simulink model "VehCtrlMdel240918_2018b"  (R2019b)
settings: Solver=FixedStepDiscrete  StartTime=0.0  StopTime=10.0  FixedStep=0.0005  RelTol=1e-3  EnableMultiTasking=on
values from neighbouring files (symbols this model uses):
  Ax_OffSet = 0.0    [VehCtrlMdelDictionary.sldd]
  Ay_OffSet = 0.0    [VehCtrlMdelDictionary.sldd]
  Caf = 460.0    [VehCtrlMdelDictionary.sldd]    (also in trqvparameter.m = 460)
  Car = 440.0    [VehCtrlMdelDictionary.sldd]    (also in trqvparameter.m = 440)
  dwf = 1.2    [VehCtrlMdelDictionary.sldd]    (also in trqvparameter.m)
  dwr = 1.2    [VehCtrlMdelDictionary.sldd]    (also in trqvparameter.m)
  h = 0.29    [VehCtrlMdelDictionary.sldd]    (also in trqvparameter.m)
  i1 = 11.4    [VehCtrlMdelDictionary.sldd]    (also in trqvparameter.m)
  i2 = 3.4    [VehCtrlMdelDictionary.sldd]    (also in trqvparameter.m)
  Iz = 105.0    [VehCtrlMdelDictionary.sldd]    (also in trqvparameter.m = 105)
  Kc = 1.0    [VehCtrlMdelDictionary.sldd]    (also in trqvparameter.m = 10)
  Ki = 1.0    [VehCtrlMdelDictionary.sldd]    (also in trqvparameter.m = 20)
  Kp = 2.0    [VehCtrlMdelDictionary.sldd]    (also in trqvparameter.m = 30)
  Ldwf = 1.2    [VehCtrlMdelDictionary.sldd]    (also in trqvparameter.m)
  Ldwr = 1.16    [VehCtrlMdelDictionary.sldd]    (also in trqvparameter.m)
  lf = 0.761    [VehCtrlMdelDictionary.sldd]    (also in trqvparameter.m)
  lr = 0.831    [VehCtrlMdelDictionary.sldd]    (also in trqvparameter.m)
  m = 340.0    [VehCtrlMdelDictionary.sldd]    (also in trqvparameter.m = 340)
  Offset_Angle = 0.0    [VehCtrlMdelDictionary.sldd]
  Qa = 0.1    [VehCtrlMdelDictionary.sldd]    (also in trqvparameter.m)
  Ra = 2.0    [VehCtrlMdelDictionary.sldd]    (also in trqvparameter.m = 2)
  Rt = 0.2    [VehCtrlMdelDictionary.sldd]    (also in trqvparameter.m)
  thr1 = 2.0    [VehCtrlMdelDictionary.sldd]    (also in trqvparameter.m = 2)
  thr2 = 0.5    [VehCtrlMdelDictionary.sldd]    (also in trqvparameter.m)
  thr3 = 0.8    [VehCtrlMdelDictionary.sldd]    (also in trqvparameter.m)
  thr4 = 0.5    [VehCtrlMdelDictionary.sldd]    (also in trqvparameter.m)
  thr5 = -0.5    [VehCtrlMdelDictionary.sldd]    (also in trqvparameter.m)
  TrqRquRate = 0.1    [VehCtrlMdelDictionary.sldd]    (also in trqvparameter.m)
  YawRate_OffSet = 0.0    [VehCtrlMdelDictionary.sldd]
undefined symbols (not defined in the file or in its folder): DiscIntNeverNeededParam, I_AN07_5V, I_AN08_5V, I_AN09_5V, I_AN10_5V, I_SW01_L, I_SW02_L, I_SW03_L, O_SW12_HS1A, O_SW14_HS1A, PWM3
libraries: simulink x144, ec5744lib x68, canmsglib x18
(part 3 of 5)

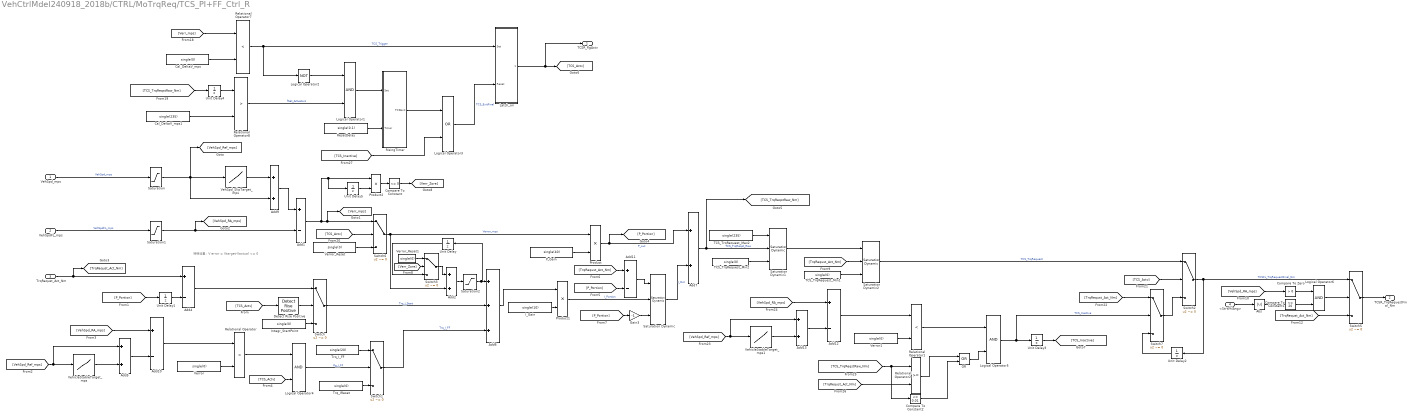
== system VehCtrlMdel240918_2018b/CTRL/MoTrqReq/TCS_PI+FF_Ctrl_R ==
  note: 特殊设置：V error = Vtarget-Vactual <= 0
  VehSpd_mps : Inport
  VehSpdFL_mps : Inport  Port=2
  TrqRequst_Act_Nm : Inport  Port=3
  <StrWhlAng> : Inport  Port=4
  Abs : Abs
  Add{1,4,10..12} (5 alike) : Sum  Inputs=+-
  Add{2,5,7,9,13} (5 alike) : Sum
  Add6 : Sum  Inputs=+++
  Cal_DeltaV_mps : Constant  Value=single(0)
  Cal_DeltaV_mps1 : Constant  Value=single(235)
  Compare To Constant : simulink/Logic and Bit Operations/Compare To Constant  relop=<=  const=0  OutDataTypeStr=boolean
  Compare To Constant1 : simulink/Logic and Bit Operations/Compare To Constant  relop=<=  const=20  OutDataTypeStr=boolean
  Compare To Constant2 : simulink/Logic and Bit Operations/Compare To Constant  relop=<=  const=0.01  OutDataTypeStr=boolean
  Compare To Zero : simulink/Logic and Bit Operations/Compare To Zero  relop=>  OutDataTypeStr=boolean
  Detect Rise Positive : simulink/Logic and Bit Operations/Detect Rise Positive  vinit=0  OutDataTypeStr=boolean
  Gain3 : Gain  Gain=-1
  I_Gain : Constant  Value=single(10)
  Integr_StartPoint : Constant  Value=single(0)
  Latch_on : Subsystem
  Logical Operator{1,4..6} (4 alike) : Logic  AllPortsSameDT=off  OutDataTypeStr=boolean
  Logical Operator2 : Logic  Operator=NOT  AllPortsSameDT=off  OutDataTypeStr=boolean
  Logical Operator3 : Logic  Operator=OR  AllPortsSameDT=off  OutDataTypeStr=boolean
  OR : Logic  Operator=OR  AllPortsSameDT=off  OutDataTypeStr=boolean
  P_Gain : Constant  Value=single(40)
  Product : Product
  Product1 : Product
  Product2 : Product
  Relational Operator : RelationalOperator  Operator=<  OutDataTypeStr=boolean  RndMeth=Simplest
  Relational Operator1 : RelationalOperator  Operator=<  OutDataTypeStr=boolean  RndMeth=Simplest
  Relational Operator2 : RelationalOperator  OutDataTypeStr=boolean  RndMeth=Simplest
  Relational Operator7 : RelationalOperator  Operator=<  OutDataTypeStr=boolean  RndMeth=Simplest
  Relational Operator8 : RelationalOperator  Operator=>  OutDataTypeStr=boolean  RndMeth=Simplest
  ResetDelay : Constant  Value=single(0.1)
  RisingTimer : Subsystem
  Saturation : Saturate  UpperLimit=40  LowerLimit=0
  Saturation Dynamic : simulink/Discontinuities/Saturation Dynamic  OutMin=[]  OutMax=[]  OutDataTypeStr=Inherit: Same as second input  OutDataType=fixdt(1, 16)  OutScaling=2^-10  DoSatur=off
  Saturation Dynamic1 : simulink/Discontinuities/Saturation Dynamic  OutMin=[]  OutMax=[]  OutDataTypeStr=Inherit: Same as second input  OutDataType=fixdt(1, 16)  OutScaling=2^-10  DoSatur=off
  Saturation Dynamic2 : simulink/Discontinuities/Saturation Dynamic  OutMin=[]  OutMax=[]  OutDataTypeStr=Inherit: Same as second input  OutDataType=fixdt(1, 16)  OutScaling=2^-10  DoSatur=off
  Saturation1 : Saturate  UpperLimit=50  LowerLimit=0
  Saturation2 : Saturate  UpperLimit=400  LowerLimit=-100
  Switch{,1..3,5..7} (7 alike) : Switch  Criteria=u2 ~= 0
  TCS_TrqRequest_Max2 : Constant  Value=single(235)
  TCS_TrqRequest_Min1 : Constant  Value=single(0)
  TCS_TrqRequest_Min2 : Constant  Value=single(0)
  Trq_IReset : Constant  Value=single(0)
  Trq_I_FF : Constant  Value=single(20)
  Unit Delay{,1..5} (6 alike) : UnitDelay  SampleTime=-1  HasFrameUpgradeWarning=on
  VehSpd_SlipTarget_mps : Lookup_n-D  NumberOfTableDimensions=1  BreakpointsForDimension1=[0,3,25,30]  Table=[0.3,0.3,2.5,2.5]  ExtrapMethod=Clip  InternalRulePriority=Speed  RndMeth=Simplest  InputSameDT=on
  VehicleStableTarget_mps : Lookup_n-D  NumberOfTableDimensions=1  BreakpointsForDimension1=[0,3,25,30]  Table=[0.4,0.4,1.2,1.2]  ExtrapMethod=Clip  InternalRulePriority=Speed  RndMeth=Simplest  InputSameDT=on
  VehicleStableTarget_mps1 : Lookup_n-D  NumberOfTableDimensions=1  BreakpointsForDimension1=[0,3,25,30]  Table=[0.4,0.4,1.2,1.2]  ExtrapMethod=Clip  InternalRulePriority=Speed  RndMeth=Simplest  InputSameDT=on
  Verror : Constant  Value=single(0)
  Verror1 : Constant  Value=single(0)
  Verror_Reset : Constant  Value=single(0)
  Verror_Reset1 : Constant  Value=single(0)
  TCSR_flgActv : Outport
  TCSR_TrqRequestFinal_Nm : Outport  Port=2
  wires:
  Add1/1 -> Unit Delay5/1, Product2/1, Switch6/1, [Verr_mps]
  Switch2/1 -> Switch5/1, Unit Delay2/1  "TCSFL_TrqRequestFinal_Nm"
  Saturation/1 -> Add9/2, VehSpd_SlipTarget_mps/1, [VehSpd_Ref_mps]
  Gain3/1 -> Saturation Dynamic/3
  [P_Portion] -> Gain3/1
  P_Gain/1 -> Product/2
  Unit Delay/1 -> Switch3/3
  Add2/1 -> Saturation2/1
  [TrqRequst_Act_Nm] -> Add11/1
  Saturation2/1 -> Unit Delay/1, Add6/1
  Switch/1 -> Add6/2  "Trq_I_Start"
  Saturation Dynamic/1 -> Add7/2  "I_Out"
  VehSpd_mps/1 -> Saturation/1  "VehSpd_mps"
  Saturation1/1 -> Add1/2, [VehSpd_RA_mps]
  Product1/1 -> Saturation Dynamic/2  "I_Portion"
  TrqRequst_Act_Nm/1 -> Add4/1, [TrqRequst_Act_Nm]
  Add6/1 -> Product1/1
  TCS_TrqRequest_Min1/1 -> Saturation Dynamic2/3
  Detect Rise Positive/1 -> Switch/2
  Integr_StartPoint/1 -> Switch/3
  I_Gain/1 -> Product1/2
  Saturation Dynamic2/1 -> Switch2/1  "TCS_TrqRequest"
  Add7/1 -> Saturation Dynamic1/2, [TCS_TrqReqstRaw_Nm]  "TCS_TrqReqst_Raw"
  [TrqRequst_Act_Nm] -> Saturation Dynamic2/2
  VehSpd_SlipTarget_mps/1 -> Add9/1
  Add9/1 -> Add1/1
  [Verr_mps] -> Relational Operator7/1
  Cal_DeltaV_mps/1 -> Relational Operator7/2
  Relational Operator7/1 -> Latch_on/1(Set), Logical Operator2/1  "TCS_Trigger"
  [TCS_TrqReqstRaw_Nm] -> Unit Delay4/1
  Logical Operator2/1 -> Logical Operator1/1
  Relational Operator8/1 -> Logical Operator1/2  "fSat_Actuators"
  Cal_DeltaV_mps1/1 -> Relational Operator8/2
  Logical Operator1/1 -> RisingTimer/1(Set)
  ResetDelay/1 -> RisingTimer/2(Timer)
  RisingTimer/1(TCSExit) -> Logical Operator3/1
  Logical Operator3/1 -> Latch_on/2(Reset)  "TCS_ExitFinal"
  Latch_on/1(flg_TCSActv) -> TCSR_flgActv/1, [TCS_Actv]
  [TCS_Actv] -> Switch6/2
  Verror_Reset/1 -> Switch6/3
  Switch6/1 -> Product/1, Add2/2  "Verror_mps"
  Product/1 -> [P_Portion], Add7/1  "P_out"
  [TCS_Actv] -> Detect Rise Positive/1
  [P_Portion] -> Unit Delay1/1
  Add4/1 -> Switch/1
  Unit Delay1/1 -> Add4/2
  [VehSpd_Ref_mps] -> Add5/1, VehicleStableTarget_mps/1
  VehicleStableTarget_mps/1 -> Add5/2
  Add5/1 -> Add10/2
  [VehSpd_RA_mps] -> Add10/1
  Add10/1 -> Relational Operator/1
  Verror/1 -> Relational Operator/2
  Relational Operator/1 -> Logical Operator4/1
  [TCS_Actv] -> Logical Operator4/2
  Logical Operator4/1 -> Switch1/2  "flg_I_FF"
  Trq_I_FF/1 -> Switch1/1
  Trq_IReset/1 -> Switch1/3
  Switch1/1 -> Add6/3  "Trq_I_FF"
  [P_Portion] -> Add11/2
  Add11/1 -> Saturation Dynamic/1
  [TCS_Actv] -> Switch2/2
  Switch7/1 -> Switch2/3
  [TrqRequst_Act_Nm] -> Switch7/1
  Verror1/1 -> Relational Operator1/2
  Add12/1 -> Relational Operator1/1
  [VehSpd_RA_mps] -> Add12/1
  Add13/1 -> Add12/2
  VehicleStableTarget_mps1/1 -> Add13/2
  [VehSpd_Ref_mps] -> VehicleStableTarget_mps1/1, Add13/1
  [TCS_TrqReqstRaw_Nm] -> Compare To Constant2/1, Relational Operator2/1
  [TrqRequst_Act_Nm] -> Relational Operator2/2
  Relational Operator1/1 -> Logical Operator5/1
  Relational Operator2/1 -> OR/1
  Logical Operator5/1 -> Unit Delay3/1, Switch7/2  "TCS_Inactive"
  Unit Delay3/1 -> [TCS_Inactive]
  [TCS_Inactive] -> Logical Operator3/2
  Unit Delay4/1 -> Relational Operator8/1
  VehSpdFL_mps/1 -> Saturation1/1  "VehSpdFL_mps"
  Saturation Dynamic1/1 -> Saturation Dynamic2/1
  TCS_TrqRequest_Max2/1 -> Saturation Dynamic1/1
  TCS_TrqRequest_Min2/1 -> Saturation Dynamic1/3
  Switch3/1 -> Add2/1
  Verror_Reset1/1 -> Switch3/1
  [Verr_Zore] -> Switch3/2
  Unit Delay5/1 -> Product2/2
  Product2/1 -> Compare To Constant/1
  Compare To Constant/1 -> [Verr_Zore]
  <StrWhlAng>/1 -> Abs/1
  Compare To Zero/1 -> Logical Operator6/1
  Abs/1 -> Compare To Constant1/1
  [VehSpd_RA_mps] -> Compare To Zero/1
  Compare To Constant1/1 -> Logical Operator6/2
  Unit Delay2/1 -> Switch7/3
  Switch5/1 -> TCSR_TrqRequestFinal_Nm/1
  Logical Operator6/1 -> Switch5/2
  [TrqRequst_Act_Nm] -> Switch5/3
  Compare To Constant2/1 -> OR/2
  OR/1 -> Logical Operator5/2

== system VehCtrlMdel240918_2018b/Input/ABS_Receive/ABS_BUS_state ==
  CANOK : Inport
  ID : Inport  Port=2
  Msg : Inport  Port=3
  function : TriggerPort  TriggerType=function-call  VariantControl=(inherit)
  Bus Creator3 : BusCreator  Inputs=4
  IMU_state : Subsystem  TreatAsAtomicUnit=on
  ABS_BUS : Outport  VectorParamsAs1DForOutWhenUnconnected=off
  wires:
  IMU_state/3(ABS_WS_FL) -> Bus Creator3/3
  IMU_state/2(ABS_WS_RL) -> Bus Creator3/2
  IMU_state/1(ABS_WS_FR) -> Bus Creator3/1
  Bus Creator3/1 -> ABS_BUS/1
  ID/1 -> IMU_state/1(ID)
  CANOK/1 -> IMU_state/Enable
  Msg/1 -> IMU_state/2(Msg)
  IMU_state/4(ABS_WS_RR) -> Bus Creator3/4

== system VehCtrlMdel240918_2018b/Input/AMKMCU_Receive/FLAMKMCU ==
  AMKMCU_state : Subsystem  TreatAsAtomicUnit=on
  AMKMCU_state1 : Subsystem  TreatAsAtomicUnit=on
  AMKMCU_state2 : Subsystem  TreatAsAtomicUnit=on
  CANReceive1 : ec5744lib/RapidECU_U3/04CANCommunication/CANReceive  canmodule=1  canbuffer=2  canmessageid=642  canmessagetype=Standard(11-bit ID)  datalength=8  sampletime=-1
      settings: SourceProductName=ECUCoder for MPC5744
  CANReceive2 : ec5744lib/RapidECU_U3/04CANCommunication/CANReceive  canmodule=1  canbuffer=3  canmessageid=644  canmessagetype=Standard(11-bit ID)  datalength=8  sampletime=-1
      settings: SourceProductName=ECUCoder for MPC5744
  CANReceive3 : ec5744lib/RapidECU_U3/04CANCommunication/CANReceive  canmodule=1  canbuffer=1  canmessageid=640  canmessagetype=Standard(11-bit ID)  datalength=8  sampletime=-1
      settings: SourceProductName=ECUCoder for MPC5744
  Terminator1 : Terminator
  Terminator2 : Terminator
  Terminator3 : Terminator
  FLAMKMCUtoVCU1 : Outport  VectorParamsAs1DForOutWhenUnconnected=off
  FLAMKMCUtoVCU2 : Outport  Port=2  VectorParamsAs1DForOutWhenUnconnected=off
  FLAMKMCUtoVCU3 : Outport  Port=3  VectorParamsAs1DForOutWhenUnconnected=off
  wires:
  CANReceive2/2 -> AMKMCU_state2/1(CANOK)
  CANReceive1/4 -> AMKMCU_state1/3(Msg)
  CANReceive3/5 -> Terminator3/1
  CANReceive1/3 -> AMKMCU_state1/2(ID)
  CANReceive1/1 -> AMKMCU_state1/Trigger
  CANReceive2/4 -> AMKMCU_state2/3(Msg)
  CANReceive3/3 -> AMKMCU_state/2(ID)
  CANReceive3/2 -> AMKMCU_state/1(CANOK)
  CANReceive2/3 -> AMKMCU_state2/2(ID)
  CANReceive1/2 -> AMKMCU_state1/1(CANOK)
  CANReceive1/5 -> Terminator1/1
  CANReceive3/4 -> AMKMCU_state/3(Msg)
  CANReceive2/5 -> Terminator2/1
  CANReceive3/1 -> AMKMCU_state/Trigger
  CANReceive2/1 -> AMKMCU_state2/Trigger
  AMKMCU_state2/1(FLAMKMCUtoVCU3) -> FLAMKMCUtoVCU3/1  "FLAMKMCUtoVCU3"
  AMKMCU_state/1(FLAMKtoVCU1) -> FLAMKMCUtoVCU1/1
  AMKMCU_state1/1(FLAMKMCUtoVCU2) -> FLAMKMCUtoVCU2/1  "FLAMKMCUtoVCU2"

== system VehCtrlMdel240918_2018b/Input/AMKMCU_Receive/FRAMKMCU ==
  AMKMCU_state : Subsystem  TreatAsAtomicUnit=on
  AMKMCU_state1 : Subsystem  TreatAsAtomicUnit=on
  AMKMCU_state2 : Subsystem  TreatAsAtomicUnit=on
  CANReceive1 : ec5744lib/RapidECU_U3/04CANCommunication/CANReceive  canmodule=1  canbuffer=5  canmessageid=643  canmessagetype=Standard(11-bit ID)  datalength=8  sampletime=-1
      settings: SourceProductName=ECUCoder for MPC5744
  CANReceive2 : ec5744lib/RapidECU_U3/04CANCommunication/CANReceive  canmodule=1  canbuffer=6  canmessageid=387  canmessagetype=Standard(11-bit ID)  datalength=8  sampletime=-1
      settings: SourceProductName=ECUCoder for MPC5744
  CANReceive3 : ec5744lib/RapidECU_U3/04CANCommunication/CANReceive  canmodule=1  canbuffer=4  canmessageid=641  canmessagetype=Standard(11-bit ID)  datalength=8  sampletime=-1
      settings: SourceProductName=ECUCoder for MPC5744
  Terminator1 : Terminator
  Terminator2 : Terminator
  Terminator3 : Terminator
  FRAMKMCUtoVCU1 : Outport  VectorParamsAs1DForOutWhenUnconnected=off
  FRAMKMCUtoVCU2 : Outport  Port=2  VectorParamsAs1DForOutWhenUnconnected=off
  FRAMKMCUtoVCU3 : Outport  Port=3  VectorParamsAs1DForOutWhenUnconnected=off
  wires:
  AMKMCU_state1/1(FRAMKMCUtoVCU2) -> FRAMKMCUtoVCU2/1  "FRAMKMCUtoVCU2"
  AMKMCU_state/1(FRAMKMCUtoVCU1) -> FRAMKMCUtoVCU1/1  "FRAMKMCUtoVCU1"
  AMKMCU_state2/1(FRAMKMCUtoVCU3) -> FRAMKMCUtoVCU3/1  "FRAMKMCUtoVCU3"
  CANReceive2/1 -> AMKMCU_state2/Trigger
  CANReceive3/1 -> AMKMCU_state/Trigger
  CANReceive2/5 -> Terminator2/1
  CANReceive3/4 -> AMKMCU_state/3(Msg)
  CANReceive1/5 -> Terminator1/1
  CANReceive1/2 -> AMKMCU_state1/1(CANOK)
  CANReceive2/3 -> AMKMCU_state2/2(ID)
  CANReceive3/2 -> AMKMCU_state/1(CANOK)
  CANReceive3/3 -> AMKMCU_state/2(ID)
  CANReceive2/4 -> AMKMCU_state2/3(Msg)
  CANReceive1/1 -> AMKMCU_state1/Trigger
  CANReceive1/3 -> AMKMCU_state1/2(ID)
  CANReceive3/5 -> Terminator3/1
  CANReceive1/4 -> AMKMCU_state1/3(Msg)
  CANReceive2/2 -> AMKMCU_state2/1(CANOK)

== system VehCtrlMdel240918_2018b/Input/BMS_Recive/ABS_BUS_state ==
  CANOK : Inport
  ID : Inport  Port=2
  Msg : Inport  Port=3
  function : TriggerPort  TriggerType=function-call  VariantControl=(inherit)
  Bus Creator : BusCreator  Inputs=9
  IMU_state : Subsystem  TreatAsAtomicUnit=on
  BMS_BUS : Outport  VectorParamsAs1DForOutWhenUnconnected=off
  wires:
  Bus Creator/1 -> BMS_BUS/1
  ID/1 -> IMU_state/1(ID)
  CANOK/1 -> IMU_state/Enable
  Msg/1 -> IMU_state/2(Msg)
  IMU_state/1(BatAlmlv) -> Bus Creator/1
  IMU_state/2(BatLife) -> Bus Creator/2
  IMU_state/3(BatState) -> Bus Creator/3
  IMU_state/4(LSBAz) -> Bus Creator/4
  IMU_state/5(LSBVz) -> Bus Creator/5
  IMU_state/6(MSBAz) -> Bus Creator/6
  IMU_state/7(MSBVz) -> Bus Creator/7
  IMU_state/8(SOCz) -> Bus Creator/8
  IMU_state/9(SOHz) -> Bus Creator/9

== system VehCtrlMdel240918_2018b/Input/EMRAXMCU_RECIEVE/MCU_pwr ==
  CANOK : Inport
  ID : Inport  Port=2
  Msg : Inport  Port=3
  function : TriggerPort  TriggerType=function-call  VariantControl=(inherit)
  Bus Creator3 : BusCreator  Inputs=5
  MCU_VCUMeter1 : Subsystem  TreatAsAtomicUnit=on
  MCU_pwr : Outport
  wires:
  Bus Creator3/1 -> MCU_pwr/1
  Msg/1 -> MCU_VCUMeter1/2(Msg)
  CANOK/1 -> MCU_VCUMeter1/Enable
  ID/1 -> MCU_VCUMeter1/1(ID)
  MCU_VCUMeter1/1("AC_current ") -> Bus Creator3/1  "AC_current"
  MCU_VCUMeter1/2(MCU_temp) -> Bus Creator3/2  "MCU_temp"
  MCU_VCUMeter1/3(current) -> Bus Creator3/3  "current"
  MCU_VCUMeter1/4(motor_temp) -> Bus Creator3/4  "motor_temp"
  MCU_VCUMeter1/5(voltage) -> Bus Creator3/5  "voltage"

== system VehCtrlMdel240918_2018b/Input/EMRAXMCU_RECIEVE/MCU_state ==
  CANOK : Inport
  ID : Inport  Port=2
  Msg : Inport  Port=3
  function : TriggerPort  TriggerType=function-call  VariantControl=(inherit)
  Bus Creator3 : BusCreator  Inputs=15
  MCU_state : Subsystem  TreatAsAtomicUnit=on
  Out1 : Outport  VectorParamsAs1DForOutWhenUnconnected=off
  wires:
  Msg/1 -> MCU_state/2(Msg)
  CANOK/1 -> MCU_state/Enable
  ID/1 -> MCU_state/1(ID)
  Bus Creator3/1 -> Out1/1
  MCU_state/1(12V_error) -> Bus Creator3/1
  MCU_state/2(alarm) -> Bus Creator3/2
  MCU_state/3(undervol) -> Bus Creator3/3
  MCU_state/4(controller_ready) -> Bus Creator3/4
  MCU_state/5(MCU_temp_warn) -> Bus Creator3/5
  MCU_state/6(mode_cmd8) -> Bus Creator3/6
  MCU_state/7(motor_temp_warn) -> Bus Creator3/7
  MCU_state/8(overcur) -> Bus Creator3/8
  MCU_state/9(pow_lim_warn) -> Bus Creator3/9
  MCU_state/10(overvol) -> Bus Creator3/10
  MCU_state/11(precharge) -> Bus Creator3/11
  MCU_state/12(rotation_warn) -> Bus Creator3/12
  MCU_state/13(selfcech) -> Bus Creator3/13
  MCU_state/14(RPM) -> Bus Creator3/14
  MCU_state/15(torque) -> Bus Creator3/15

== system VehCtrlMdel240918_2018b/Input/IMU_Recieve/IMU_state ==
  CANOK : Inport
  ID : Inport  Port=2
  Msg : Inport  Port=3
  function : TriggerPort  TriggerType=function-call  VariantControl=(inherit)
  Bus Creator3 : BusCreator  Inputs=7
  MCU_state : Subsystem  TreatAsAtomicUnit=on
  MeaModule1 : ec5744lib/RapidECU_U3/07Calibration/MeaModule  signal=IMU_Ax_Value
      settings: SourceProductName=ECUCoder for MPC5744
  IMU_BUS : Outport  VectorParamsAs1DForOutWhenUnconnected=off
  wires:
  Msg/1 -> MCU_state/2(Msg)
  CANOK/1 -> MCU_state/Enable
  ID/1 -> MCU_state/1(ID)
  Bus Creator3/1 -> IMU_BUS/1
  MeaModule1/1 -> Bus Creator3/1
  MCU_state/2(IMU_Ay_Value) -> Bus Creator3/2  "IMU_Ay_Value"
  MCU_state/3(IMU_Yaw_Value) -> Bus Creator3/3  "IMU_Yaw_Value"
  MCU_state/4(IMU_Ay_Valid) -> Bus Creator3/4  "IMU_Ay_Valid"
  MCU_state/5(IMU_DTC) -> Bus Creator3/5  "IMU_DTC"
  MCU_state/6(IMU_Yaw_Valid) -> Bus Creator3/6  "IMU_Yaw_Valid"
  MCU_state/7(IMU_Ax_Valid) -> Bus Creator3/7  "IMU_Ax_Valid"
  MCU_state/1(IMU_Ax_Value) -> MeaModule1/1  "IMU_Ax_Value"

== system VehCtrlMdel240918_2018b/Input/StrSnis_Receive/StrWhSnis_state ==
  CANOK : Inport
  ID : Inport  Port=2
  Msg : Inport  Port=3
  function : TriggerPort  TriggerType=function-call  VariantControl=(inherit)
  Bus Creator3 : BusCreator  Inputs=3
  IMU_state : Subsystem  TreatAsAtomicUnit=on
  IMU_BUS : Outport  VectorParamsAs1DForOutWhenUnconnected=off
  wires:
  Msg/1 -> IMU_state/2(Msg)
  CANOK/1 -> IMU_state/Enable
  ID/1 -> IMU_state/1(ID)
  Bus Creator3/1 -> IMU_BUS/1
  IMU_state/1(StrWhlAng) -> Bus Creator3/1  "StrWhlAng"
  IMU_state/2(StrWhlAngV) -> Bus Creator3/2  "StrWhlAngV"
  IMU_state/3(StrWhlAngAliveRollCnt) -> Bus Creator3/3  "StrWhlAngAliveRollCnt"

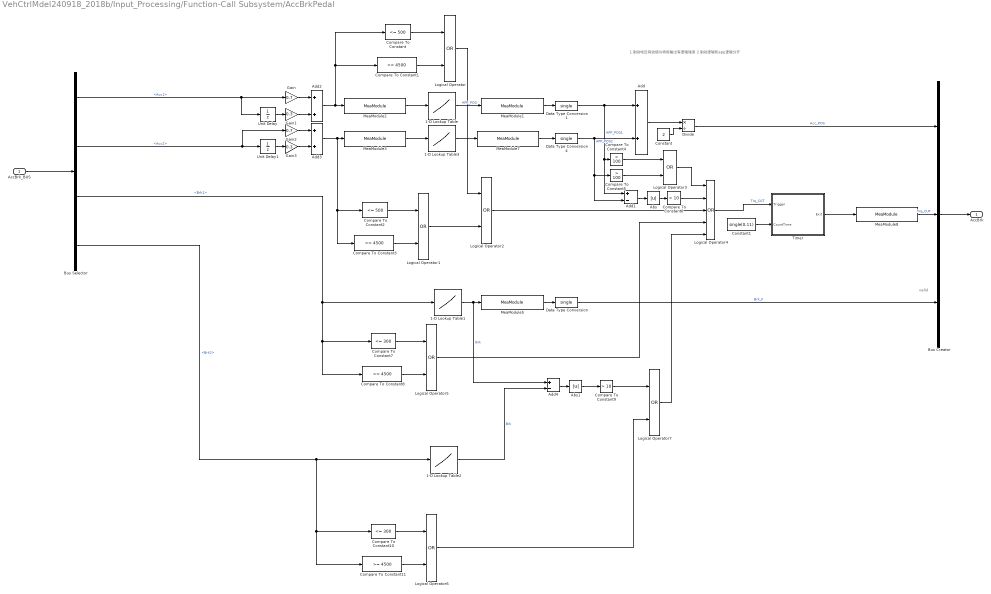
== system VehCtrlMdel240918_2018b/Input_Processing/Function-Call Subsystem/AccBrkPedal ==
  note: 1.制动电压有效值与转矩输出有逻辑错误
      | 2.制动逻辑和app逻辑分开
  note: valid
  AccBrk_BUS : Inport
  1-D Lookup Table : Lookup_n-D  NumberOfTableDimensions=1  BreakpointsForDimension1=single([1330,1590]);  BreakpointsForDimension1DataTypeStr=single  Table=single([0,100]);  TableDataTypeStr=single  ExtrapMethod=Clip  InternalRulePriority=Speed  RndMeth=Simplest  InputSameDT=on
  1-D Lookup Table1 : Lookup_n-D  NumberOfTableDimensions=1  BreakpointsForDimension1=single([500,4500]);  BreakpointsForDimension1DataTypeStr=single  Table=single([0,10000]);  TableDataTypeStr=single  ExtrapMethod=Clip  InternalRulePriority=Speed  RndMeth=Simplest  InputSameDT=on
  1-D Lookup Table2 : Lookup_n-D  NumberOfTableDimensions=1  BreakpointsForDimension1=single([500,4500]);  BreakpointsForDimension1DataTypeStr=single  Table=single([0,10000]);  TableDataTypeStr=single  ExtrapMethod=Clip  InternalRulePriority=Speed  RndMeth=Simplest  InputSameDT=on
  1-D Lookup Table3 : Lookup_n-D  NumberOfTableDimensions=1  BreakpointsForDimension1=single([2324,2600]);  BreakpointsForDimension1DataTypeStr=single  Table=single([0,100]);  TableDataTypeStr=single  ExtrapMethod=Clip  InternalRulePriority=Speed  RndMeth=Simplest  InputSameDT=on
  Abs : Abs
  Abs1 : Abs
  Add : Sum
  Add1 : Sum  Inputs=+-
  Add2 : Sum
  Add3 : Sum
  Add4 : Sum  Inputs=+-
  Bus Selector : BusSelector  OutputSignals=Acc1,Acc2,Brk1,Brk2
  Bus Creator : BusCreator  Inputs=3
  Compare To Constant : simulink/Logic and Bit Operations/Compare To Constant  relop=<=  const=500  OutDataTypeStr=boolean
  Compare To Constant{1,3,8,11} (4 alike) : simulink/Logic and Bit Operations/Compare To Constant  relop=>=  const=4500  OutDataTypeStr=boolean
  Compare To Constant10 : simulink/Logic and Bit Operations/Compare To Constant  relop=<=  const=300  OutDataTypeStr=boolean
  Compare To Constant2 : simulink/Logic and Bit Operations/Compare To Constant  relop=<=  const=500  OutDataTypeStr=boolean
  Compare To Constant4 : simulink/Logic and Bit Operations/Compare To Constant  relop=>  const=100  OutDataTypeStr=boolean
  Compare To Constant5 : simulink/Logic and Bit Operations/Compare To Constant  relop=>  const=100  OutDataTypeStr=boolean
  Compare To Constant6 : simulink/Logic and Bit Operations/Compare To Constant  relop=>  const=10  OutDataTypeStr=boolean
  Compare To Constant7 : simulink/Logic and Bit Operations/Compare To Constant  relop=<=  const=300  OutDataTypeStr=boolean
  Compare To Constant9 : simulink/Logic and Bit Operations/Compare To Constant  relop=>  const=10  OutDataTypeStr=boolean
  Constant : Constant  Value=2
  Constant1 : Constant  Value=single(0.11)
  Data Type Conversion : DataTypeConversion  OutDataTypeStr=single
  Data Type Conversion1 : DataTypeConversion  OutDataTypeStr=single
  Data Type Conversion4 : DataTypeConversion  OutDataTypeStr=single
  Divide : Product  Inputs=*/  OutDataTypeStr=single
  Gain : Gain  Gain=0.7
  Gain1 : Gain  Gain=0.3
  Gain2 : Gain  Gain=0.7
  Gain3 : Gain  Gain=0.3
  Logical Operator{,1..3,5..7} (7 alike) : Logic  Operator=OR  AllPortsSameDT=off  OutDataTypeStr=boolean
  Logical Operator4 : Logic  Operator=OR  Inputs=5  AllPortsSameDT=off  OutDataTypeStr=boolean
  MeaModule1 : ec5744lib/RapidECU_U3/07Calibration/MeaModule  signal=Acc_POS1
      settings: SourceProductName=ECUCoder for MPC5744
  MeaModule2 : ec5744lib/RapidECU_U3/07Calibration/MeaModule  signal=Acc_vol
      settings: SourceProductName=ECUCoder for MPC5744
  MeaModule3 : ec5744lib/RapidECU_U3/07Calibration/MeaModule  signal=Acc_vol2
      settings: SourceProductName=ECUCoder for MPC5744
  MeaModule5 : ec5744lib/RapidECU_U3/07Calibration/MeaModule  signal=F_BrkPrs
      settings: SourceProductName=ECUCoder for MPC5744
  MeaModule7 : ec5744lib/RapidECU_U3/07Calibration/MeaModule  signal=Acc_POS2
      settings: SourceProductName=ECUCoder for MPC5744
  MeaModule8 : ec5744lib/RapidECU_U3/07Calibration/MeaModule  signal=Trq_CUT
      settings: SourceProductName=ECUCoder for MPC5744
  Timer : Stateflow chart  TreatAsAtomicUnit=on
  Unit Delay : UnitDelay  SampleTime=-1  HasFrameUpgradeWarning=on
  Unit Delay1 : UnitDelay  SampleTime=-1  HasFrameUpgradeWarning=on
  AccBrk : Outport  VectorParamsAs1DForOutWhenUnconnected=off
  wires:
  AccBrk_BUS/1 -> Bus Selector/1
  Bus Selector/1 -> Unit Delay/1, Gain/1  "<Acc1>"
  Bus Selector/3 -> 1-D Lookup Table1/1, Compare To Constant7/1, Compare To Constant8/1  "<Brk1>"
  Bus Selector/2 -> Gain2/1, Unit Delay1/1  "<Acc2>"
  Gain/1 -> Add2/1
  Compare To Constant6/1 -> Logical Operator4/2
  Compare To Constant5/1 -> Logical Operator3/2
  Compare To Constant4/1 -> Logical Operator3/1
  Logical Operator3/1 -> Logical Operator4/1
  Unit Delay1/1 -> Gain3/1
  1-D Lookup Table/1 -> MeaModule1/1  "APP_POS"
  Gain3/1 -> Add3/2
  Add/1 -> Divide/1
  Logical Operator1/1 -> Logical Operator2/2
  Compare To Constant8/1 -> Logical Operator5/2
  Logical Operator4/1 -> Timer/1(Trigger)  "Trq_CUT"
  Logical Operator5/1 -> Logical Operator4/4
  Compare To Constant3/1 -> Logical Operator1/2
  Compare To Constant1/1 -> Logical Operator/2
  Add2/1 -> Compare To Constant/1, Compare To Constant1/1, MeaModule2/1
  Gain2/1 -> Add3/1
  Add3/1 -> Compare To Constant3/1, Compare To Constant2/1, MeaModule3/1
  1-D Lookup Table3/1 -> MeaModule7/1
  Compare To Constant7/1 -> Logical Operator5/1
  Data Type Conversion1/1 -> Add1/1, Compare To Constant4/1, Add/1  "APP_POS1"
  MeaModule8/1 -> Bus Creator/2  "Trq_CUT"
  Divide/1 -> Bus Creator/1  "Acc_POS"
  Compare To Constant/1 -> Logical Operator/1
  Constant/1 -> Divide/2
  Data Type Conversion4/1 -> Add1/2, Compare To Constant5/1, Add/2  "APP_POS2"
  MeaModule5/1 -> Data Type Conversion/1
  MeaModule3/1 -> 1-D Lookup Table3/1
  Logical Operator2/1 -> Logical Operator4/3
  Data Type Conversion/1 -> Bus Creator/3  "Brk_F"
  MeaModule2/1 -> 1-D Lookup Table/1
  Gain1/1 -> Add2/2
  Add1/1 -> Abs/1
  Abs/1 -> Compare To Constant6/1
  MeaModule7/1 -> Data Type Conversion4/1
  Compare To Constant2/1 -> Logical Operator1/1
  MeaModule1/1 -> Data Type Conversion1/1
  Logical Operator/1 -> Logical Operator2/1
  1-D Lookup Table1/1 -> Add4/1, MeaModule5/1  "Brk"
  Unit Delay/1 -> Gain1/1
  Bus Creator/1 -> AccBrk/1
  Timer/1(Exit) -> MeaModule8/1
  Constant1/1 -> Timer/2(CountTime)
  Bus Selector/4 -> Compare To Constant11/1, Compare To Constant10/1, 1-D Lookup Table2/1  "<Brk2>"
  1-D Lookup Table2/1 -> Add4/2  "Brk"
  Compare To Constant11/1 -> Logical Operator6/2
  Compare To Constant10/1 -> Logical Operator6/1
  Logical Operator6/1 -> Logical Operator7/2
  Add4/1 -> Abs1/1
  Abs1/1 -> Compare To Constant9/1
  Compare To Constant9/1 -> Logical Operator7/1
  Logical Operator7/1 -> Logical Operator4/5

== system VehCtrlMdel240918_2018b/Input_Processing/Function-Call Subsystem/IMU ==
  IMU : Inport
  Bus Selector : BusSelector  OutputSignals=IMU_Ax_Value,IMU_Ay_Value,IMU_Yaw_Value,IMU_Ay_Valid,IMU_DTC,IMU_Yaw_Valid,IMU_Ax_Valid
  Bus Creator : BusCreator  Inputs=7
  Subsystem : Subsystem
  g_mpss : Gain  Gain=9.8
  g_mpss1 : Gain  Gain=9.8
  IMU_BUS : Outport  VectorParamsAs1DForOutWhenUnconnected=off
  wires:
  IMU/1 -> Bus Selector/1
  Bus Selector/4 -> Bus Creator/4  "<IMU_Ay_Valid>"
  Bus Selector/5 -> Bus Creator/5  "<IMU_DTC>"
  Bus Selector/6 -> Bus Creator/6  "<IMU_Yaw_Valid>"
  Bus Selector/7 -> Bus Creator/7  "<IMU_Ax_Valid>"
  Bus Selector/1 -> g_mpss/1  "<IMU_Ax_Value>"
  Bus Selector/2 -> g_mpss1/1  "<IMU_Ay_Value>"
  Bus Creator/1 -> IMU_BUS/1
  g_mpss/1 -> Subsystem/1(IMU_Ax_Value)
  g_mpss1/1 -> Subsystem/2(IMU_Ay_Value)
  Bus Selector/3 -> Subsystem/3(IMU_Yaw_Value)  "<IMU_Yaw_Value>"
  Subsystem/1(IMU_Ax_Value_out) -> Bus Creator/1
  Subsystem/2(IMU_Ay_Value_out) -> Bus Creator/2
  Subsystem/3(IMU_Yaw_Value_out) -> Bus Creator/3

== system VehCtrlMdel240918_2018b/Input_Processing/Function-Call Subsystem/SWAS ==
  SWAS : Inport
  1-D Lookup Table : Lookup_n-D  NumberOfTableDimensions=1  BreakpointsForDimension1=|  Table=|  InternalRulePriority=Speed  RndMeth=Simplest  InputSameDT=on
      BreakpointsForDimension1=|
      | single([-119.993
      | -109.997
      | -100
      | -90.0034
      | -80.0067
      | -69.9933
      | -59.9966
      | -50
      | -40.0034
      | -30.0067
      | -19.9933
      | -9.99664
      | 0
      | 9.99664
      | 19.9933
      | 30.0067
      | 40.0034
      | 50
      | 59.9966
      | 69.9933
      | 80.0067
      | 90.0034
      | 100
      | 109.997
      | ]);
      Table=|
      | single([-26.072928
      | -23.62248
      | -20.834568
      | -18.002448
      | -15.197904
      | -12.620232
      | -10.131048
      | -8.139672
      | -6.2976672
      | -4.605012
      | -3.0893688
      | -1.4907528
      | -0.07467624
      | 1.40778
      | 2.9621448
      | 4.7211768
      | 6.5521152
      | 8.737056
      | 10.944144
      | 13.743144
      | 17.25012
      | 20.375424
      | 24.070536
      | 27.505584
      | ]);
  1-D Lookup Table1 : Lookup_n-D  NumberOfTableDimensions=1  BreakpointsForDimension1=|  Table=|  InternalRulePriority=Speed  RndMeth=Simplest  InputSameDT=on
      BreakpointsForDimension1=|
      | single([-119.995
      | -109.993
      | -99.9916
      | -90.0067
      | -80.005
      | -70.0034
      | -60.0017
      | -50
      | -39.9983
      | -29.9966
      | -19.995
      | -9.99328
      | 0.00840477
      | 9.99328
      | 19.995
      | 29.9966
      | 39.9983
      | 50
      | 60.0017
      | 70.0034
      | 80.005
      | 90.0067
      | 100.008
      | 109.993
      | ]);
      Table=|
      | single([-26.816256
      | -23.524848
      | -19.851048
      | -16.282584
      | -13.40676
      | -10.314792
      | -7.65504
      | -5.3554968
      | -3.4548912
      | -1.5044184
      | 0.02493504
      | 1.4379192
      | 2.8675296
      | 4.2638976
      | 5.76
      | 7.35588
      | 9.101304
      | 11.04624
      | 12.94128
      | 15.35724
      | 18.244152
      | 20.937168
      | 23.630112
      | 26.306496
      | ]);
  Abs : Abs
  Add1 : Sum
  Add2 : Sum
  Bus Selector : BusSelector  OutputSignals=StrWhlAng,StrWhlAngV
  Bus Creator : BusCreator  Inputs=5
  Compare To Constant : simulink/Logic and Bit Operations/Compare To Constant  relop=>  const=120  OutDataTypeStr=boolean
  Constant1 : Constant  Value=single(1200)
  Constant2 : Constant  Value=single(1200)
  Constant3 : Constant  Value=single(-1200)
  Constant4 : Constant  Value=single(-1200)
  Constant5 : Constant  Value=single(0.11)
  Gain : Gain  Gain=0.7
  Gain1 : Gain  Gain=0.3
  Gain2 : Gain  Gain=0.7
  Gain3 : Gain  Gain=0.3
  NOT : Logic  Operator=NOT  AllPortsSameDT=off  OutDataTypeStr=boolean
  Rate Limiter Dynamic : simulink/Discontinuities/Rate Limiter Dynamic
      settings: SourceProductName=Simulink
  Rate Limiter Dynamic1 : simulink/Discontinuities/Rate Limiter Dynamic
      settings: SourceProductName=Simulink
  Saturation1 : Saturate  UpperLimit=1200  LowerLimit=0
  Timer : Stateflow chart  TreatAsAtomicUnit=on
  Unit Delay : UnitDelay  SampleTime=-1  HasFrameUpgradeWarning=on
  Unit Delay1 : UnitDelay  SampleTime=-1  HasFrameUpgradeWarning=on
  StrWhlAng&V : Outport  VectorParamsAs1DForOutWhenUnconnected=off
  wires:
  SWAS/1 -> Bus Selector/1
  Bus Selector/2 -> Rate Limiter Dynamic1/2  "<StrWhlAngV>"
  Constant3/1 -> Rate Limiter Dynamic/3
  Constant2/1 -> Rate Limiter Dynamic/1
  Gain/1 -> Add2/1
  Gain1/1 -> Add2/2
  Rate Limiter Dynamic/1 -> Abs/1, Gain/1, Unit Delay/1
  Unit Delay/1 -> Gain1/1
  Add2/1 -> 1-D Lookup Table1/1, Bus Creator/4, 1-D Lookup Table/1  "StrWhlAng"
  Bus Creator/1 -> StrWhlAng&V/1
  Add1/1 -> Bus Creator/5  "StrWhlAngV"
  Rate Limiter Dynamic1/1 -> Saturation1/1
  Bus Selector/1 -> Rate Limiter Dynamic/2  "<StrWhlAng>"
  Constant1/1 -> Rate Limiter Dynamic1/1
  Constant4/1 -> Rate Limiter Dynamic1/3
  1-D Lookup Table/1 -> Bus Creator/2  "FLWhlStrAng"
  1-D Lookup Table1/1 -> Bus Creator/3  "FRWhlStrAng"
  Unit Delay1/1 -> Gain3/1
  Gain3/1 -> Add1/2
  Gain2/1 -> Add1/1
  Saturation1/1 -> Unit Delay1/1, Gain2/1  "StrWhlAngV"
  Abs/1 -> Compare To Constant/1
  NOT/1 -> Bus Creator/1  "WhlStrAng_Valid"
  Constant5/1 -> Timer/2(CountTime)
  Compare To Constant/1 -> Timer/1(Trigger)  "WhlStrAng_Valid"
  Timer/1(Exit) -> NOT/1

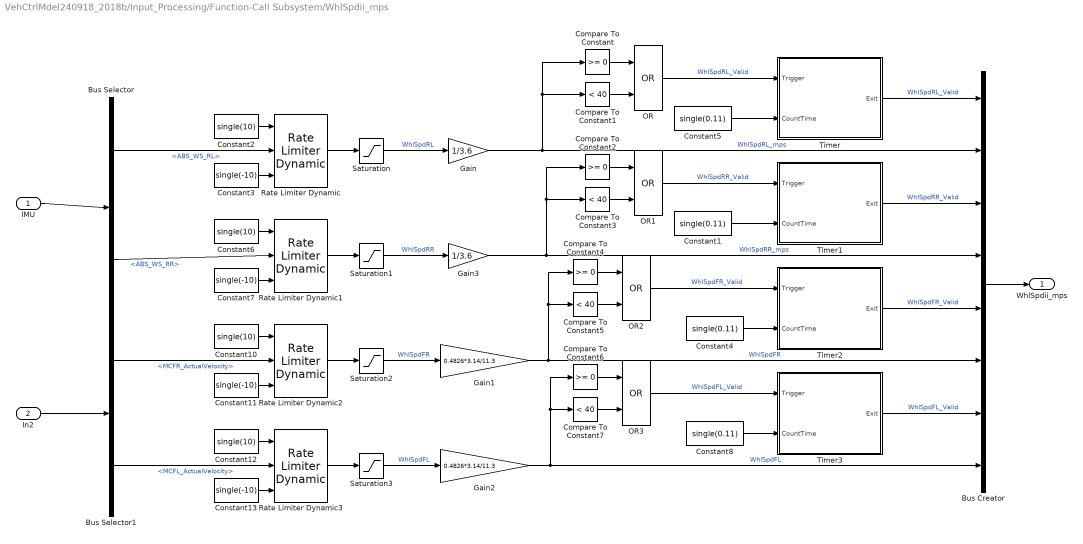
== system VehCtrlMdel240918_2018b/Input_Processing/Function-Call Subsystem/WhlSpdii_mps ==
  IMU : Inport
  In2 : Inport  Port=2
  Bus Selector : BusSelector  OutputSignals=ABS_WS_RL,ABS_WS_RR
  Bus Selector1 : BusSelector  OutputSignals=FRAMKMCUtoVCU1.MCFR_ActualVelocity,FLAMKMCUtoVCU1.MCFL_ActualVelocity
  Bus Creator : BusCreator  Inputs=8
  Compare To Constant{,2,4,6} (4 alike) : simulink/Logic and Bit Operations/Compare To Constant  relop=>=  const=0  OutDataTypeStr=boolean
  Compare To Constant{1,3,5,7} (4 alike) : simulink/Logic and Bit Operations/Compare To Constant  relop=<  const=40  OutDataTypeStr=boolean
  Constant{1,4..5,8} (4 alike) : Constant  Value=single(0.11)
  Constant{2,6,10,12} (4 alike) : Constant  Value=single(10)
  Constant{3,7,11,13} (4 alike) : Constant  Value=single(-10)
  Gain : Gain  Gain=1/3.6
  Gain1 : Gain  Gain=0.4826*3.14/11.3
  Gain2 : Gain  Gain=0.4826*3.14/11.3
  Gain3 : Gain  Gain=1/3.6
  OR{,1..3} (4 alike) : Logic  Operator=OR  AllPortsSameDT=off  OutDataTypeStr=boolean
  Rate Limiter Dynamic{,1..3} (4 alike) : simulink/Discontinuities/Rate Limiter Dynamic
      settings: SourceProductName=Simulink
  Saturation{,1..3} (4 alike) : Saturate  UpperLimit=30  LowerLimit=0
  Timer : Stateflow chart  TreatAsAtomicUnit=on
  Timer1 : Stateflow chart  TreatAsAtomicUnit=on
  Timer2 : Stateflow chart  TreatAsAtomicUnit=on
  Timer3 : Stateflow chart  TreatAsAtomicUnit=on
  WhlSpdii_mps : Outport  VectorParamsAs1DForOutWhenUnconnected=off
  wires:
  IMU/1 -> Bus Selector/1
  Bus Selector/1 -> Rate Limiter Dynamic/2  "<ABS_WS_RL>"
  Bus Selector/2 -> Rate Limiter Dynamic1/2  "<ABS_WS_RR>"
  Constant2/1 -> Rate Limiter Dynamic/1
  Constant3/1 -> Rate Limiter Dynamic/3
  Constant7/1 -> Rate Limiter Dynamic1/3
  Constant6/1 -> Rate Limiter Dynamic1/1
  Constant10/1 -> Rate Limiter Dynamic2/1
  Constant11/1 -> Rate Limiter Dynamic2/3
  Bus Selector1/1 -> Rate Limiter Dynamic2/2  "<MCFR_ActualVelocity>"
  Bus Selector1/2 -> Rate Limiter Dynamic3/2  "<MCFL_ActualVelocity>"
  Constant13/1 -> Rate Limiter Dynamic3/3
  Constant12/1 -> Rate Limiter Dynamic3/1
  In2/1 -> Bus Selector1/1
  Rate Limiter Dynamic/1 -> Saturation/1
  Rate Limiter Dynamic1/1 -> Saturation1/1
  Rate Limiter Dynamic2/1 -> Saturation2/1
  Rate Limiter Dynamic3/1 -> Saturation3/1
  Saturation/1 -> Gain/1  "WhlSpdRL"
  Saturation1/1 -> Gain3/1  "WhlSpdRR"
  Saturation2/1 -> Gain1/1  "WhlSpdFR"
  Saturation3/1 -> Gain2/1  "WhlSpdFL"
  Bus Creator/1 -> WhlSpdii_mps/1
  Gain2/1 -> Compare To Constant6/1, Compare To Constant7/1, Bus Creator/8  "WhlSpdFL"
  Gain1/1 -> Compare To Constant5/1, Compare To Constant4/1, Bus Creator/6  "WhlSpdFR"
  Gain/1 -> Compare To Constant/1, Compare To Constant1/1, Bus Creator/2  "WhlSpdRL_mps"
  Gain3/1 -> Compare To Constant2/1, Compare To Constant3/1, Bus Creator/4  "WhlSpdRR_mps"
  Compare To Constant/1 -> OR/1
  Compare To Constant1/1 -> OR/2
  Compare To Constant3/1 -> OR1/2
  Compare To Constant2/1 -> OR1/1
  Compare To Constant4/1 -> OR2/1
  Compare To Constant5/1 -> OR2/2
  Compare To Constant7/1 -> OR3/2
  Compare To Constant6/1 -> OR3/1
  Timer/1(Exit) -> Bus Creator/1  "WhlSpdRL_Valid"
  Timer1/1(Exit) -> Bus Creator/3  "WhlSpdRR_Valid"
  Timer2/1(Exit) -> Bus Creator/5  "WhlSpdFR_Valid"
  Timer3/1(Exit) -> Bus Creator/7  "WhlSpdFL_Valid"
  Constant5/1 -> Timer/2(CountTime)
  OR/1 -> Timer/1(Trigger)  "WhlSpdRL_Valid"
  OR1/1 -> Timer1/1(Trigger)  "WhlSpdRR_Valid"
  Constant1/1 -> Timer1/2(CountTime)
  Constant4/1 -> Timer2/2(CountTime)
  OR2/1 -> Timer2/1(Trigger)  "WhlSpdFR_Valid"
  Constant8/1 -> Timer3/2(CountTime)
  OR3/1 -> Timer3/1(Trigger)  "WhlSpdFL_Valid"

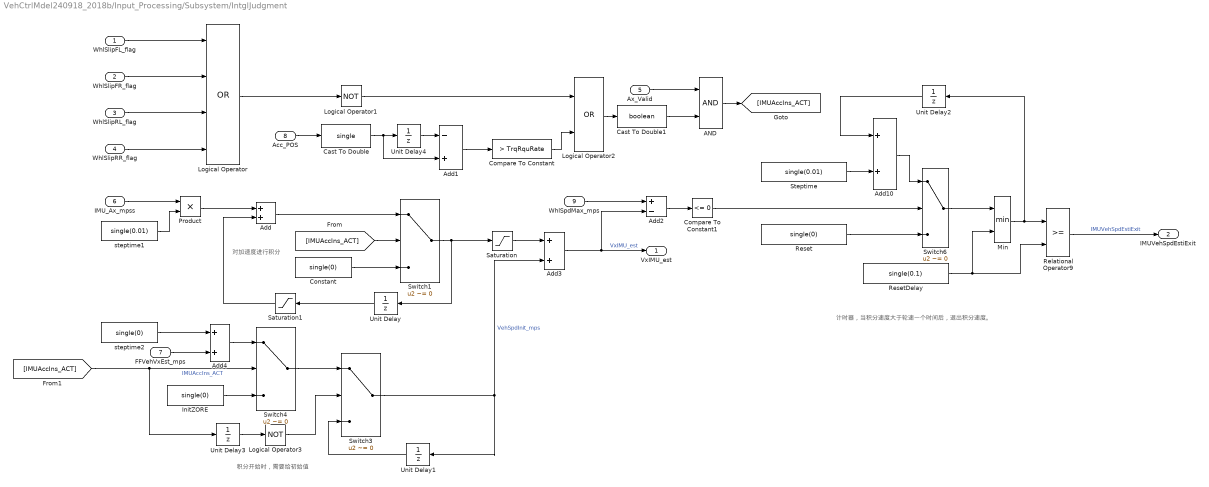
== system VehCtrlMdel240918_2018b/Input_Processing/Subsystem/IntglJudgment  ==
  note: 对加速度进行积分
  note: 计时器，当积分速度大于轮速一个时间后，退出积分速度。
  note: 积分开始时，需要给初始值
  WhlSlipFL_flag : Inport
  WhlSlipFR_flag : Inport  Port=2
  WhlSlipRL_flag : Inport  Port=3
  WhlSlipRR_flag : Inport  Port=4
  Ax_Valid : Inport  Port=5
  IMU_Ax_mpss : Inport  Port=6
  FFVehVxEst_mps : Inport  Port=7
  Acc_POS : Inport  Port=8
  WhlSpdMax_mps : Inport  Port=9
  AND : Logic  AllPortsSameDT=off  OutDataTypeStr=boolean
  Add{,3..4,10} (4 alike) : Sum
  Add1 : Sum  Inputs=-+
  Add2 : Sum  Inputs=+-
  Cast To Double : DataTypeConversion  OutDataTypeStr=single
  Cast To Double1 : DataTypeConversion  OutDataTypeStr=boolean
  Compare To Constant : simulink/Logic and Bit Operations/Compare To Constant  relop=>  const=TrqRquRate  OutDataTypeStr=boolean
  Compare To Constant1 : simulink/Logic and Bit Operations/Compare To Constant  relop=<=  const=0  OutDataTypeStr=boolean
  Constant : Constant  Value=single(0)
  InitZORE : Constant  Value=single(0)
  Logical Operator : Logic  Operator=OR  Inputs=4  AllPortsSameDT=off  OutDataTypeStr=boolean
  Logical Operator1 : Logic  Operator=NOT  AllPortsSameDT=off  OutDataTypeStr=boolean
  Logical Operator2 : Logic  Operator=OR  AllPortsSameDT=off  OutDataTypeStr=boolean
  Logical Operator3 : Logic  Operator=NOT  AllPortsSameDT=off  OutDataTypeStr=boolean
  Min : MinMax  Inputs=2
  Product : Product
  Relational Operator9 : RelationalOperator  OutDataTypeStr=boolean  RndMeth=Simplest
  Reset : Constant  Value=single(0)
  ResetDelay : Constant  Value=single(0.1)
  Saturation : Saturate  UpperLimit=200  LowerLimit=-10
  Saturation1 : Saturate  UpperLimit=200  LowerLimit=-10
  Steptime : Constant  Value=single(0.01)
  Switch{1,3..4,6} (4 alike) : Switch  Criteria=u2 ~= 0
  Unit Delay{,1..4} (5 alike) : UnitDelay  SampleTime=-1  HasFrameUpgradeWarning=on
  steptime1 : Constant  Value=single(0.01)
  steptime2 : Constant  Value=single(0)
  VxIMU_est : Outport
  IMUVehSpdEstiExit : Outport  Port=2
  wires:
  WhlSlipFL_flag/1 -> Logical Operator/1
  WhlSlipFR_flag/1 -> Logical Operator/2
  WhlSlipRL_flag/1 -> Logical Operator/3
  WhlSlipRR_flag/1 -> Logical Operator/4
  Logical Operator/1 -> Logical Operator1/1
  Unit Delay/1 -> Saturation1/1
  Add/1 -> Switch1/1
  Constant/1 -> Switch1/3
  Logical Operator1/1 -> Logical Operator2/1
  Acc_POS/1 -> Cast To Double/1
  Unit Delay4/1 -> Add1/1
  Add1/1 -> Compare To Constant/1
  Compare To Constant/1 -> Logical Operator2/2
  [IMUAccIns_ACT] -> Switch1/2
  Logical Operator2/1 -> Cast To Double1/1
  Add2/1 -> Compare To Constant1/1
  WhlSpdMax_mps/1 -> Add2/1
  Saturation1/1 -> Add/2
  Product/1 -> Add/1
  IMU_Ax_mpss/1 -> Product/1
  steptime1/1 -> Product/2
  Saturation/1 -> Add3/1
  Add3/1 -> Add2/2, VxIMU_est/1  "VxIMU_est"
  Switch6/1 -> Min/1
  ResetDelay/1 -> Relational Operator9/2, Min/2
  Compare To Constant1/1 -> Switch6/2
  Add10/1 -> Switch6/1
  Steptime/1 -> Add10/2
  Min/1 -> Relational Operator9/1, Unit Delay2/1
  Reset/1 -> Switch6/3
  Unit Delay2/1 -> Add10/1
  Unit Delay3/1 -> Logical Operator3/1
  InitZORE/1 -> Switch4/3
  Logical Operator3/1 -> Switch3/2
  Switch3/1 -> Add3/2, Unit Delay1/1  "VehSpdInit_mps"
  Switch4/1 -> Switch3/1
  Cast To Double/1 -> Unit Delay4/1, Add1/2
  [IMUAccIns_ACT] -> Unit Delay3/1, Switch4/2  "IMUAccIns_ACT"
  Relational Operator9/1 -> IMUVehSpdEstiExit/1  "IMUVehSpdEstiExit"
  Cast To Double1/1 -> AND/2
  Unit Delay1/1 -> Switch3/3
  Add4/1 -> Switch4/1
  FFVehVxEst_mps/1 -> Add4/2
  steptime2/1 -> Add4/1
  Switch1/1 -> Saturation/1, Unit Delay/1
  AND/1 -> [IMUAccIns_ACT]
  Ax_Valid/1 -> AND/1

== system VehCtrlMdel240918_2018b/Input_Processing/Subsystem/WhlSlpageJudgment ==
  note: 实践中很难同时满足这三个条件。
      | 一般只满足后两个其中一个即可。
  note: 更改记录：1、理了信号线，更整齐。
      | 2、加速度差，加速度差的微分的判断加入滤波模块。
      | 3、轮速选取改为选取最大轮速。
  note: 选取一个最大轮速
  Vxii_mps : Inport
  IMU_YawRate_dps : Inport  Port=2
  IMU_Aa_mpss : Inport  Port=3
  VehSpdEstiZ1_mps : Inport  Port=4
  In5 : Inport  Port=5
  Bus Selector : BusSelector  OutputSignals=VxFL_mps,VxFR_mps,VxRL_mps,VxRR_mps
  Cast To Double{,1..3} (4 alike) : DataTypeConversion  OutDataTypeStr=boolean
  Constant{1..4} (4 alike) : Constant  Value=single(0.11)
  Logical Operator : Logic  Operator=OR  AllPortsSameDT=off  OutDataTypeStr=boolean
  Logical Operator1 : Logic  AllPortsSameDT=off  OutDataTypeStr=boolean
  Min1 : MinMax  Function=max  Inputs=4
  Mux : Mux
  Mux1 : Mux
  Mux2 : Mux
  Selector : Selector  InputPortWidth=4  IndexOptions=Index vector (dialog)  Indices=[1]  OutputSizes=1
  Selector1 : Selector  InputPortWidth=4  IndexOptions=Index vector (dialog)  Indices=[2]  OutputSizes=1
  Selector2 : Selector  InputPortWidth=4  IndexOptions=Index vector (dialog)  Indices=[3]  OutputSizes=1
  Selector3 : Selector  InputPortWidth=4  IndexOptions=Index vector (dialog)  Indices=[4]  OutputSizes=1
  Terminator : Terminator
  Timer : Stateflow chart  TreatAsAtomicUnit=on
  Timer1 : Stateflow chart  TreatAsAtomicUnit=on
  Timer2 : Stateflow chart  TreatAsAtomicUnit=on
  Timer3 : Stateflow chart  TreatAsAtomicUnit=on
  加速度差判断 : Subsystem
  加速度差的微分的判断 : Subsystem
  速差判断 : Subsystem
  WhlSlipFLValid_flag : Outport
  WhlSlipFRValid_flag : Outport  Port=2
  WhlSlipRLValid_flag : Outport  Port=3
  WhlSlipRRValid_flag : Outport  Port=4
  WhlSpdMax_mps : Outport  Port=5
  wires:
  Selector3/1 -> Cast To Double3/1
  Selector2/1 -> Cast To Double2/1
  [IMU_Aa_mpsss] -> 加速度差的微分的判断/5(IMU_Ax_mpss)
  [VehSpdEstiZ1_mps] -> 速差判断/5(VehSpd_mps)
  Bus Selector/3 -> 加速度差的微分的判断/3(<VxRL_mps>), Min1/3, 速差判断/3(<VxRL_mps>), 加速度差判断/3(<VxRL_mps>)  "<VxRL_mps>"
  Selector1/1 -> Cast To Double1/1
  [IMU_Aa_mpsss] -> 加速度差判断/5(IMU_Ax_mpss)
  Bus Selector/4 -> 加速度差判断/4(<VxRR_mps>), Min1/4, 速差判断/4(<VxRR_mps>), 加速度差的微分的判断/4(<VxRR_mps>)  "<VxRR_mps>"
  IMU_YawRate_dps/1 -> [IMU_YawRate_dps]
  Vxii_mps/1 -> Bus Selector/1
  Bus Selector/1 -> 加速度差的微分的判断/1(<VxFL_mps>), 加速度差判断/1(<VxFL_mps>), Min1/1, 速差判断/1(<VxFL_mps>)  "<VxFL_mps>"
  VehSpdEstiZ1_mps/1 -> [VehSpdEstiZ1_mps]
  Selector/1 -> Cast To Double/1
  Bus Selector/2 -> 加速度差的微分的判断/2(<VxFR_mps>), 加速度差判断/2(<VxFR_mps>), Min1/2, 速差判断/2(<VxFR_mps>)  "<VxFR_mps>"
  IMU_Aa_mpss/1 -> [IMU_Aa_mpsss]
  [IMU_YawRate_dps] -> Terminator/1
  Timer/1(Exit) -> WhlSlipFLValid_flag/1  "WhlSlipFLValid_flag"
  Cast To Double2/1 -> Timer2/1(Trigger)  "WhlSlipRLValid_flag"
  Cast To Double3/1 -> Timer3/1(Trigger)  "WhlSlipRRValid_flag"
  速差判断/1(y) -> Mux/1  "速差"
  速差判断/2(y1) -> Mux/2
  速差判断/3(y2) -> Mux/3
  速差判断/4(y3) -> Mux/4
  加速度差判断/1(y) -> Mux1/1  "加速度差"
  加速度差判断/2(y1) -> Mux1/2
  加速度差判断/3(y2) -> Mux1/3
  加速度差判断/4(y3) -> Mux1/4
  加速度差的微分的判断/1(y) -> Mux2/1  "加速度差的微分"
  加速度差的微分的判断/2(y1) -> Mux2/2
  加速度差的微分的判断/3(y2) -> Mux2/3
  加速度差的微分的判断/4(y3) -> Mux2/4
  Mux1/1 -> Logical Operator/1
  Mux2/1 -> Logical Operator/2
  Mux/1 -> Logical Operator1/1
  Logical Operator/1 -> Logical Operator1/2
  Logical Operator1/1 -> Selector3/1, Selector2/1, Selector1/1, Selector/1
  Min1/1 -> WhlSpdMax_mps/1
  In5/1 -> 速差判断/6(In6)
  Constant1/1 -> Timer/2(CountTime)
  Cast To Double/1 -> Timer/1(Trigger)  "WhlSlipFLValid_flag"
  Timer1/1(Exit) -> WhlSlipFRValid_flag/1  "WhlSlipFRValid_flag"
  Cast To Double1/1 -> Timer1/1(Trigger)  "WhlSlipFRValid_flag"
  Timer2/1(Exit) -> WhlSlipRLValid_flag/1  "WhlSlipRLValid_flag"
  Timer3/1(Exit) -> WhlSlipRRValid_flag/1  "WhlSlipRRValid_flag"
  Constant2/1 -> Timer1/2(CountTime)
  Constant3/1 -> Timer2/2(CountTime)
  Constant4/1 -> Timer3/2(CountTime)
